simulink model "ballonbeam_matlab1"  (R2025b)
settings: Solver=VariableStepAuto  StartTime=0.0  StopTime=6.562  RelTol=1e-3
values from neighbouring files (symbols this model uses):
  K_d = 11.9318    [parametry_reg.m]    (also in regulacja_porownanie.m)
  K_t = K_rad*pi/180    (= 20.5460159545)    [parametry_reg.m]    (also in regulacja_porownanie.m)
  Kd = Kd_STM*Ts    (= 0.1628)    [parametry_reg.m]    (also in regulacja_porownanie.m = 0.1408)
  Ki = Ki_STM/Ts    (= 0.172972972973)    [parametry_reg.m]    (also in regulacja_porownanie.m = 0.2)
  Kp = Kp_STM    (= 0.26)    [parametry_reg.m]    (also in regulacja_porownanie.m)
  T_serw = 0.095    [parametry_reg.m]    (also in regulacja_porownanie.m)
  Ts = 0.037    [parametry_reg.m]    (also in regulacja_porownanie.m = 0.032)
settings Model: Creator=mati  LastModifiedBy=mati

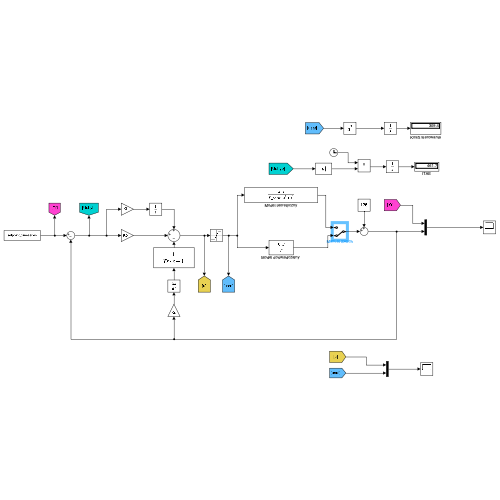
[thumbnail: Simulink's stored preview of the top-level diagram]
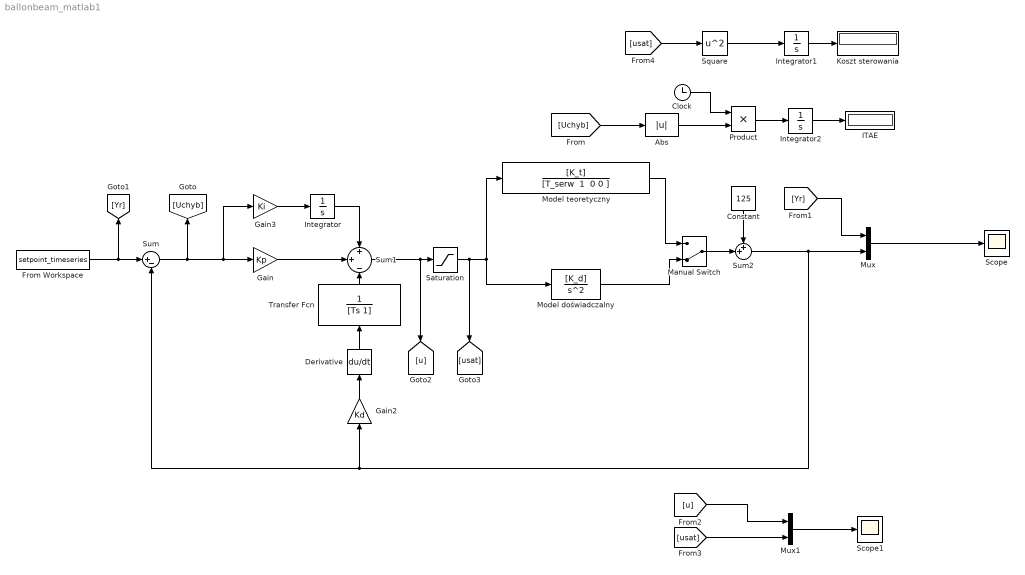
== system ballonbeam_matlab1 ==
  Abs : Abs  SaturateOnIntegerOverflow=off
  Clock : Clock
  Constant : Constant  Value=125
  Derivative : Derivative
  From Workspace : FromWorkspace  VariableName=setpoint_timeseries
  Gain : Gain  Gain=Kp
  Gain2 : Gain  Gain=Kd
  Gain3 : Gain  Gain=Ki
  ITAE : Display
  Integrator : Integrator
  Integrator1 : Integrator
  Integrator2 : Integrator
  Koszt sterowania : Display
  Manual Switch : ManualSwitch  CurrentSetting=0
  "Model doświadczalny " : TransferFcn  Numerator=[K_d]  Denominator=[1 0 0]
  Model teoretyczny : TransferFcn  Numerator=[K_t]  Denominator="[T_serw  1  0 0 ]"
  Mux : Mux  Inputs=2
  Mux1 : Mux  Inputs=2
  Product : Product
  Saturation : Saturate  UpperLimit=30  LowerLimit=-30
  Scope : Scope
      settings: ActiveDisplayYMinimum=114.84410646107965  ActiveDisplayYMaximum=216.403041850283
  Scope1 : Scope
      settings: ActiveDisplayYMinimum=-1  ActiveDisplayYMaximum=1
  Square : Math  Operator=square
  Sum : Sum  Inputs=|+-
  Sum1 : Sum  Inputs=+|+|-
  Sum2 : Sum  Inputs=++|
  Transfer Fcn : TransferFcn  Denominator=[Ts 1]
  wires:
  Gain/1 -> Sum1/2
  Sum/1 -> Gain3/1, Gain/1, [Uchyb]
  "Model doświadczalny "/1 -> Manual Switch/2
  Gain3/1 -> Integrator/1
  Gain2/1 -> Derivative/1
  Sum1/1 -> Saturation/1, [u]
  Saturation/1 -> [usat], Model teoretyczny/1, "Model doświadczalny "/1
  From Workspace/1 -> Sum/1, [Yr]
  Mux/1 -> Scope/1
  [Yr] -> Mux/1
  [usat] -> Mux1/2
  [u] -> Mux1/1
  Mux1/1 -> Scope1/1
  Abs/1 -> Product/2
  Clock/1 -> Product/1
  [Uchyb] -> Abs/1
  Product/1 -> Integrator2/1
  Integrator2/1 -> ITAE/1
  Square/1 -> Integrator1/1
  Integrator1/1 -> Koszt sterowania/1
  [usat] -> Square/1
  Integrator/1 -> Sum1/1
  Model teoretyczny/1 -> Manual Switch/1
  Derivative/1 -> Transfer Fcn/1
  Transfer Fcn/1 -> Sum1/3
  Manual Switch/1 -> Sum2/2
  Constant/1 -> Sum2/1
  Sum2/1 -> Mux/2, Sum/2, Gain2/1
